simulink model "dynamic_calib"  (Simulink 8.8)
settings: Solver=FixedStepDiscrete  StartTime=0.0  StopTime=tEnd  FixedStep=CONFIG.Ts  RelTol=1e-3  EnableMultiTasking=on
undefined symbols (not defined in the file or in its folder): calibDelta, CONFIG, tSwitch, USE_h_ONLY, USE_JOINT_VELOCITY
libraries: WBToolboxLibrary x32
settings Model: SuppressorTable=22 serialization::archive 11 0 3 0 0 0 11 0  Creator=gabri  LastModifiedBy=gnava
settings DataIOCC: SignalLoggingSaveFormat=Dataset
settings DebuggingCC: UnderspecifiedInitializationDetection=Simplified  MergeDetectMultiDrivingBlocksExec=error  SolverPrmCheckMsg=warning  FcnCallInpInsideContextMsg=error  StateNameClashWarn=none
settings GRTTargetCC: CombineOutputUpdateFcns=on  GRTInterface=off
settings ConfigComp: CovSFcnEnable=off

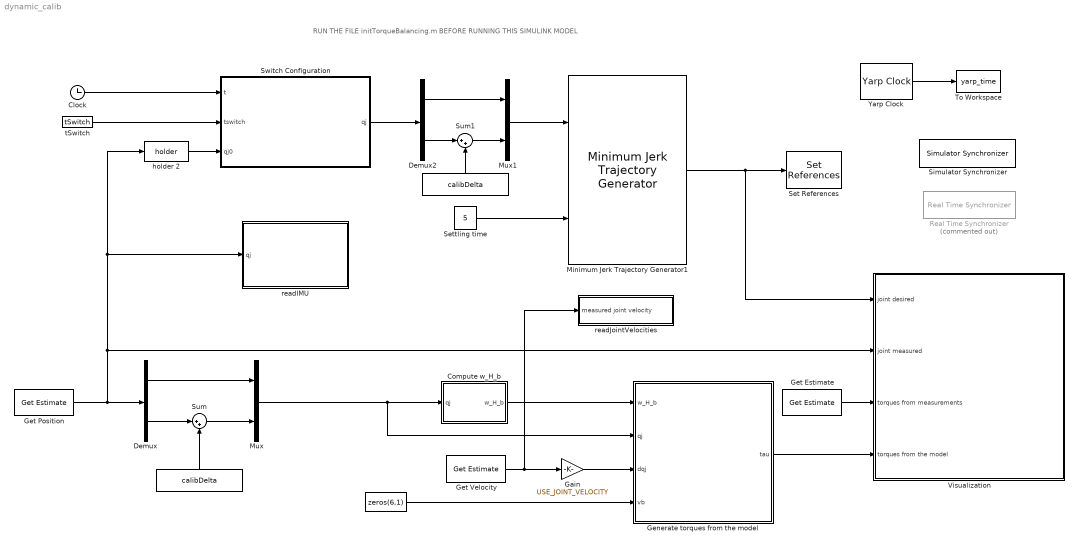
== system dynamic_calib ==
  note: RUN THE FILE initTorqueBalancing.m BEFORE RUNNING THIS SIMULINK MODEL
  "           " : Constant  Value=zeros(6,1)
  "                   " : Constant  Value=calibDelta
  "                                                      " : Constant  Value=calibDelta
  Clock : Clock
  Compute w_H_b : Subsystem
  Demux : Demux  Outputs=[13;12]
  Demux2 : Demux  Outputs=[13;12]
  Gain : Gain  Gain=USE_JOINT_VELOCITY
  Generate torques from the model : Subsystem
  Get Estimate : WBToolboxLibrary/wholeBodyStates/Get Estimate  estimateType=Joints Torque  robotName=WBT_robotName  localName=WBT_modelName  wbiFile=WBT_wbiFilename  wbiList=WBT_wbiList
  Get Position : WBToolboxLibrary/wholeBodyStates/Get Estimate  estimateType=Joints Position  robotName=WBT_robotName  localName=WBT_modelName  wbiFile=WBT_wbiFilename  wbiList=WBT_wbiList
  Get Velocity : WBToolboxLibrary/wholeBodyStates/Get Estimate  estimateType=Joints Velocity  robotName=WBT_robotName  localName=WBT_modelName  wbiFile=WBT_wbiFilename  wbiList=WBT_wbiList
  Minimum Jerk Trajectory Generator1 : WBToolboxLibrary/Utilities/Minimum Jerk Trajectory Generator  externalSettlingTime=on  settlingTime=1  sampleTime=CONFIG.Ts  resetOnSettlingTime=off  firstDerivatives=off  secondDerivatives=off  explicitInitialValue=off
  Mux : Mux  Inputs=2
  Mux1 : Mux  Inputs=2
  Real Time Synchronizer : WBToolboxLibrary/Utilities/Real Time Synchronizer  Commented=on  period=0.01
  Set References : WBToolboxLibrary/wholeBodyActuators/Set References  controlType=Position Direct  fullOrSubControl=Full  controlledJoints=''  robotName=WBT_robotName  localName=WBT_modelName  wbiFile=WBT_wbiFilename  wbiList=WBT_wbiList
  Settling time : Constant  Value=5
  Simulator Synchronizer : WBToolboxLibrary/Utilities/Simulator Synchronizer  period=0.01  serverPortName='/clock/rpc'  clientPortName='/WBT_synchronizer/rpc:o'
  Sum : Sum  Inputs=|++
  Sum1 : Sum  Inputs=|++
  Switch Configuration : MATLAB Function  TreatAsAtomicUnit=on
  To Workspace : ToWorkspace  VariableName=yarp_time  SaveFormat=Structure With Time  SampleTime=-1
  Visualization : Subsystem
  Yarp Clock : WBToolboxLibrary/Utilities/Yarp Clock
  holder 2 : WBToolboxLibrary/Utilities/holder 
  readIMU : Subsystem
  readJointVelocities : Subsystem
  tSwitch : Constant  Value=tSwitch
  wires:
  "                                                      "/1 -> Sum/2
  Get Estimate/1 -> Visualization/3(torques from measurements)
  Get Position/1 -> readIMU/1(qj), holder 2/1, Visualization/2("joint measured "), Demux/1
  Demux/2 -> Sum/1
  Demux/1 -> Mux/1
  Mux/1 -> Generate torques from the model/2(qj), Compute w_H_b/1(qj)
  Sum/1 -> Mux/2
  Settling time/1 -> Minimum Jerk Trajectory Generator1/2
  Clock/1 -> Switch Configuration/1(t)
  tSwitch/1 -> Switch Configuration/2(tswitch)
  holder 2/1 -> Switch Configuration/3(qj0)
  Get Velocity/1 -> readJointVelocities/1("measured joint velocity "), Gain/1
  "           "/1 -> Generate torques from the model/4(vb)
  Generate torques from the model/1(tau) -> Visualization/4(torques from the model)
  "                   "/1 -> Sum1/2
  Switch Configuration/1(qj) -> Demux2/1
  Demux2/2 -> Sum1/1
  Demux2/1 -> Mux1/1
  Sum1/1 -> Mux1/2
  Mux1/1 -> Minimum Jerk Trajectory Generator1/1
  Minimum Jerk Trajectory Generator1/1 -> Visualization/1(joint desired), Set References/1
  Compute w_H_b/1(w_H_b) -> Generate torques from the model/1(w_H_b)
  Gain/1 -> Generate torques from the model/3(dqj)
  Yarp Clock/1 -> To Workspace/1

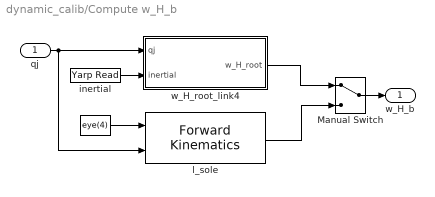
== system dynamic_calib/Compute w_H_b ==
  qj : Inport
  " " : Constant  Value=eye(4)
  Manual Switch : ManualSwitch
  inertial : WBToolboxLibrary/Utilities/Yarp Read  portName=PORTS.IMU_CALIB  signalSize=12  blocking=off  timestamp=off  autoconnect=on  errorOnConnection=on
  l_sole : WBToolboxLibrary/wholeBodyModel/Kinematics/Forward Kinematics  frameName='Waist'  robotName=WBT_robotName  localName=WBT_modelName  wbiFile=WBT_wbiFilename  wbiList=WBT_wbiList
  w_H_root_link4 : Subsystem  mask{link_name='Waist'}
      mask prompts: link_name "link name"
      mask help:
      | This block evaluates the homogeneous transformation between the world and the root link, i.e. ^wH_b. It assumes that the link specified by the variable 'link_name' has a constant position
      | w.r.t. an inertial frame, but it can rotate arbitrarily. This rotation is retrived from the IMU sensor.
      mask Display:
      | str = strrep(link_name, '_','\_');
      | port_label('output',1,['{}^{',str '}H_{root}'],'texmode','on')
      | clear str;
      | 
      | port_label('input',1,'q_j','texmode','on')
      | 
      | port_label('input',2,'inertial','texmode','on')
  w_H_b : Outport
  wires:
  qj/1 -> w_H_root_link4/1(qj), l_sole/2
  inertial/1 -> w_H_root_link4/2(inertial)
  " "/1 -> l_sole/1
  Manual Switch/1 -> w_H_b/1
  w_H_root_link4/1(w_H_root) -> Manual Switch/1
  l_sole/1 -> Manual Switch/2

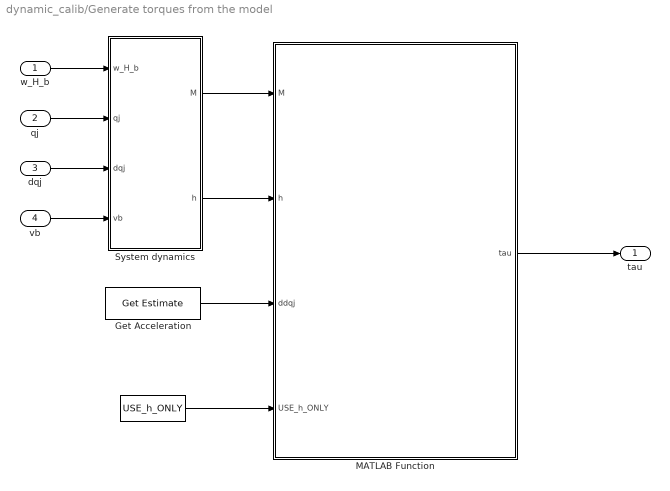
== system dynamic_calib/Generate torques from the model ==
  w_H_b : Inport
  qj : Inport  Port=2
  dqj : Inport  Port=3
  vb : Inport  Port=4
  "           " : Constant  Value=USE_h_ONLY
  Get Acceleration : WBToolboxLibrary/wholeBodyStates/Get Estimate  estimateType=Joints Acceleration  robotName=WBT_robotName  localName=WBT_modelName  wbiFile=WBT_wbiFilename  wbiList=WBT_wbiList
  MATLAB Function : MATLAB Function  TreatAsAtomicUnit=on
  System dynamics : Subsystem
  tau : Outport
  wires:
  qj/1 -> System dynamics/2(qj)
  w_H_b/1 -> System dynamics/1(w_H_b)
  MATLAB Function/1(tau) -> tau/1
  dqj/1 -> System dynamics/3(dqj)
  vb/1 -> System dynamics/4(vb)
  System dynamics/1("M ") -> MATLAB Function/1(M)
  System dynamics/2(h) -> MATLAB Function/2(h)
  Get Acceleration/1 -> MATLAB Function/3(ddqj)
  "           "/1 -> MATLAB Function/4(USE_h_ONLY)

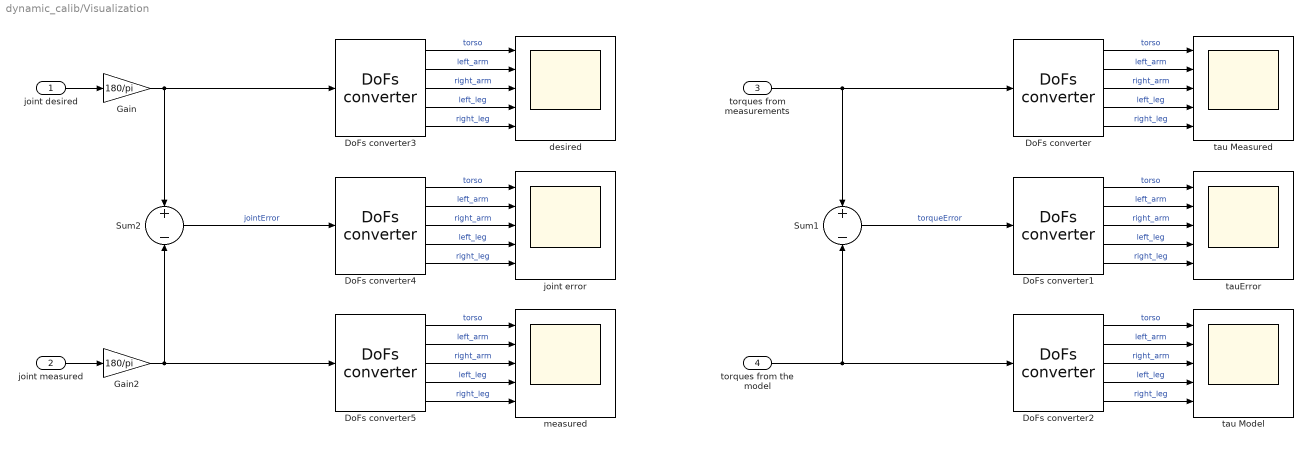
== system dynamic_calib/Visualization ==
  joint desired : Inport
  "joint measured " : Inport  Port=2
  torques from measurements : Inport  Port=3
  torques from the model : Inport  Port=4
  DoFs converter{,1..5} (6 alike) : WBToolboxLibrary/Utilities/DoFs converter  yarp2WBIOption=From WBI to YARP  robotName=WBT_robotName  localName=WBT_modelName  wbiFile=WBT_wbiFilename  wbiList=WBT_wbiList
  Gain : Gain  Gain=180/pi
  Gain2 : Gain  Gain=180/pi
  Sum1 : Sum  Inputs=+-
  Sum2 : Sum  Inputs=+-
  desired : Scope  NumInputPorts=5
  joint error : Scope  NumInputPorts=5
  measured : Scope  NumInputPorts=5
  tau Measured : Scope  NumInputPorts=5
  tau Model : Scope  NumInputPorts=5
  tauError : Scope  NumInputPorts=5
  wires:
  DoFs converter2/3 -> tau Model/3  "right_arm"
  torques from the model/1 -> DoFs converter2/1, Sum1/2
  DoFs converter/4 -> tau Measured/4  "left_leg"
  DoFs converter/3 -> tau Measured/3  "right_arm"
  DoFs converter1/5 -> tauError/5  "right_leg"
  DoFs converter1/1 -> tauError/1  "torso"
  DoFs converter1/2 -> tauError/2  "left_arm"
  DoFs converter1/4 -> tauError/4  "left_leg"
  DoFs converter1/3 -> tauError/3  "right_arm"
  Sum1/1 -> DoFs converter1/1  "torqueError"
  DoFs converter2/5 -> tau Model/5  "right_leg"
  DoFs converter2/1 -> tau Model/1  "torso"
  DoFs converter2/2 -> tau Model/2  "left_arm"
  DoFs converter2/4 -> tau Model/4  "left_leg"
  torques from measurements/1 -> DoFs converter/1, Sum1/1
  DoFs converter/5 -> tau Measured/5  "right_leg"
  DoFs converter/1 -> tau Measured/1  "torso"
  DoFs converter/2 -> tau Measured/2  "left_arm"
  DoFs converter5/3 -> measured/3  "right_arm"
  "joint measured "/1 -> Gain2/1
  DoFs converter3/4 -> desired/4  "left_leg"
  DoFs converter3/3 -> desired/3  "right_arm"
  DoFs converter4/5 -> joint error/5  "right_leg"
  DoFs converter4/1 -> joint error/1  "torso"
  DoFs converter4/2 -> joint error/2  "left_arm"
  DoFs converter4/4 -> joint error/4  "left_leg"
  DoFs converter4/3 -> joint error/3  "right_arm"
  Sum2/1 -> DoFs converter4/1  "jointError"
  DoFs converter5/5 -> measured/5  "right_leg"
  DoFs converter5/1 -> measured/1  "torso"
  DoFs converter5/2 -> measured/2  "left_arm"
  DoFs converter5/4 -> measured/4  "left_leg"
  joint desired/1 -> Gain/1
  DoFs converter3/5 -> desired/5  "right_leg"
  DoFs converter3/1 -> desired/1  "torso"
  DoFs converter3/2 -> desired/2  "left_arm"
  Gain/1 -> DoFs converter3/1, Sum2/1
  Gain2/1 -> DoFs converter5/1, Sum2/2

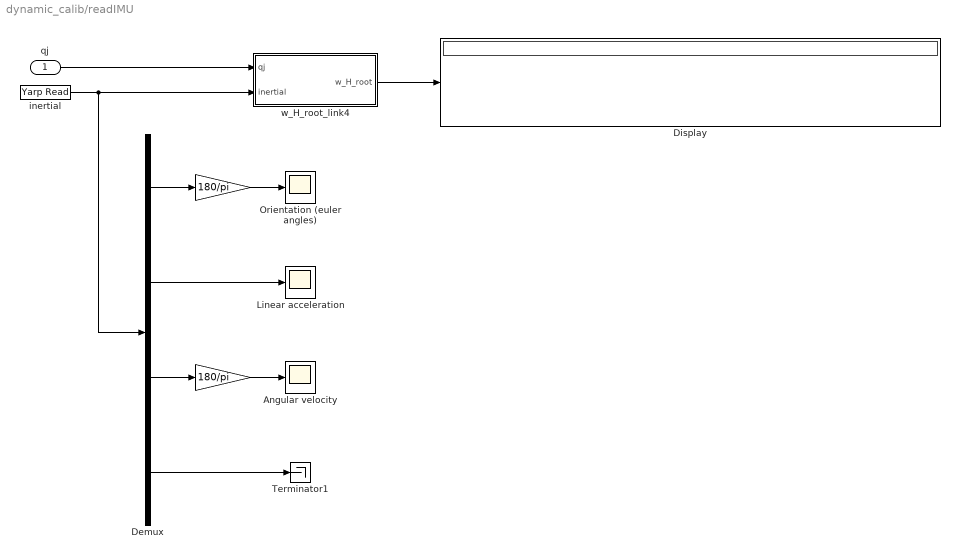
== system dynamic_calib/readIMU ==
  qj : Inport
  " " : Gain  Gain=180/pi
  "  " : Gain  Gain=180/pi
  Angular velocity : Scope
  Demux : Demux  Outputs=[3;3;3;3]
  Display : Display
  Linear acceleration : Scope
  Orientation (euler angles) : Scope
  Terminator1 : Terminator
  inertial : WBToolboxLibrary/Utilities/Yarp Read  portName=PORTS.IMU_CALIB  signalSize=12  blocking=off  timestamp=off  autoconnect=on  errorOnConnection=on
  w_H_root_link4 : Subsystem  mask{link_name='Waist'}
      mask prompts: link_name "link name"
      mask help:
      | This block evaluates the homogeneous transformation between the world and the root link, i.e. ^wH_b. It assumes that the link specified by the variable 'link_name' has a constant position
      | w.r.t. an inertial frame, but it can rotate arbitrarily. This rotation is retrived from the IMU sensor.
      mask Display:
      | str = strrep(link_name, '_','\_');
      | port_label('output',1,['{}^{',str '}H_{root}'],'texmode','on')
      | clear str;
      | 
      | port_label('input',1,'q_j','texmode','on')
      | 
      | port_label('input',2,'inertial','texmode','on')
  wires:
  qj/1 -> w_H_root_link4/1(qj)
  w_H_root_link4/1(w_H_root) -> Display/1
  Demux/1 -> "  "/1
  Demux/2 -> Linear acceleration/1
  Demux/3 -> " "/1
  inertial/1 -> w_H_root_link4/2(inertial), Demux/1
  Demux/4 -> Terminator1/1
  "  "/1 -> Orientation (euler angles)/1
  " "/1 -> Angular velocity/1

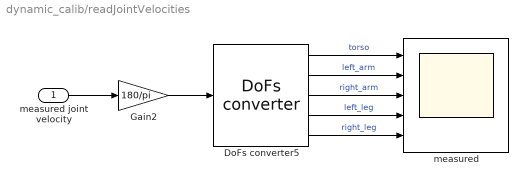
== system dynamic_calib/readJointVelocities ==
  "measured joint velocity " : Inport
  DoFs converter5 : WBToolboxLibrary/Utilities/DoFs converter  yarp2WBIOption=From WBI to YARP  robotName=WBT_robotName  localName=WBT_modelName  wbiFile=WBT_wbiFilename  wbiList=WBT_wbiList
  Gain2 : Gain  Gain=180/pi
  measured : Scope  NumInputPorts=5
  wires:
  DoFs converter5/3 -> measured/3  "right_arm"
  "measured joint velocity "/1 -> Gain2/1
  DoFs converter5/5 -> measured/5  "right_leg"
  DoFs converter5/1 -> measured/1  "torso"
  DoFs converter5/2 -> measured/2  "left_arm"
  DoFs converter5/4 -> measured/4  "left_leg"
  Gain2/1 -> DoFs converter5/1

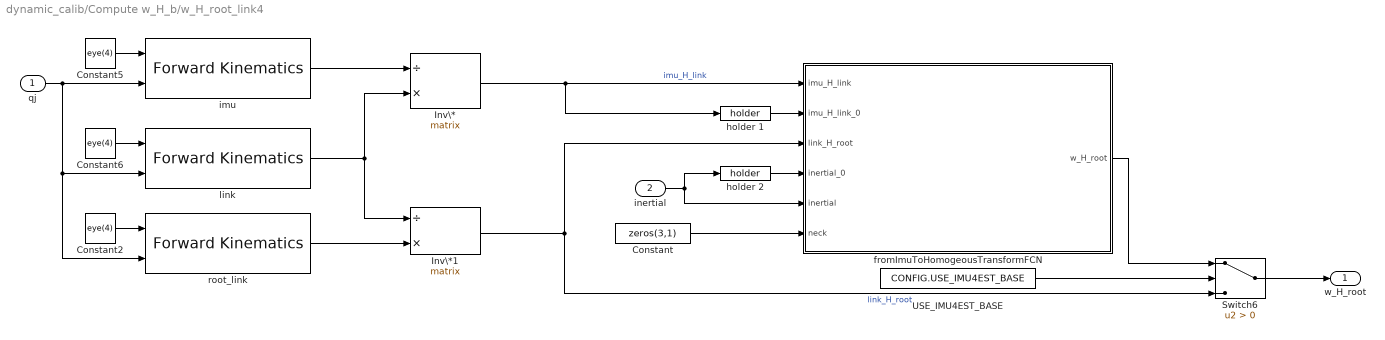
== system dynamic_calib/Compute w_H_b/w_H_root_link4 ==
  qj : Inport
  inertial : Inport  Port=2
  Constant : Constant  Value=zeros(3,1)
  Constant2 : Constant  Value=eye(4)
  Constant5 : Constant  Value=eye(4)
  Constant6 : Constant  Value=eye(4)
  Inv\* : Product  Inputs=/*  Multiplication=Matrix(*)
  Inv\*1 : Product  Inputs=/*  Multiplication=Matrix(*)
  Switch6 : Switch  Criteria=u2 > Threshold
  USE_IMU4EST_BASE : Constant  Value=CONFIG.USE_IMU4EST_BASE
  fromImuToHomogeousTransformFCN : MATLAB Function  TreatAsAtomicUnit=on
  holder 1 : WBToolboxLibrary/Utilities/holder 
  holder 2 : WBToolboxLibrary/Utilities/holder 
  imu : WBToolboxLibrary/wholeBodyModel/Kinematics/Forward Kinematics  frameName=FRAMES.IMU  robotName=WBT_robotName  localName=WBT_modelName  wbiFile=WBT_wbiFilename  wbiList=WBT_wbiList
  link : WBToolboxLibrary/wholeBodyModel/Kinematics/Forward Kinematics  frameName=link_name  robotName=WBT_robotName  localName=WBT_modelName  wbiFile=WBT_wbiFilename  wbiList=WBT_wbiList
  root_link : WBToolboxLibrary/wholeBodyModel/Kinematics/Forward Kinematics  frameName=FRAMES.BASE  robotName=WBT_robotName  localName=WBT_modelName  wbiFile=WBT_wbiFilename  wbiList=WBT_wbiList
  w_H_root : Outport
  wires:
  Constant5/1 -> imu/1
  Inv\*/1 -> holder 1/1, fromImuToHomogeousTransformFCN/1(imu_H_link)  "imu_H_link"
  imu/1 -> Inv\*/1
  Constant6/1 -> link/1
  Inv\*1/1 -> Switch6/3, fromImuToHomogeousTransformFCN/3(link_H_root)  "link_H_root"
  link/1 -> Inv\*/2, Inv\*1/1
  inertial/1 -> holder 2/1, fromImuToHomogeousTransformFCN/5(inertial)
  Switch6/1 -> w_H_root/1
  USE_IMU4EST_BASE/1 -> Switch6/2
  fromImuToHomogeousTransformFCN/1(w_H_root) -> Switch6/1
  Constant2/1 -> root_link/1
  qj/1 -> root_link/2, link/2, imu/2
  root_link/1 -> Inv\*1/2
  holder 1/1 -> fromImuToHomogeousTransformFCN/2(imu_H_link_0)
  holder 2/1 -> fromImuToHomogeousTransformFCN/4(inertial_0)
  Constant/1 -> fromImuToHomogeousTransformFCN/6(neck)

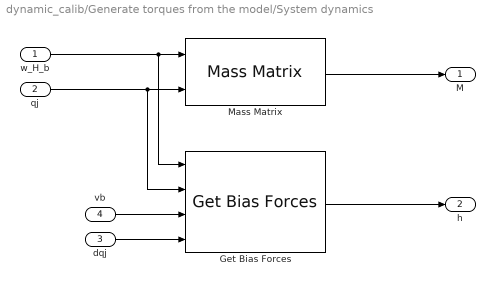
== system dynamic_calib/Generate torques from the model/System dynamics ==
  w_H_b : Inport
  qj : Inport  Port=2
  dqj : Inport  Port=3
  vb : Inport  Port=4
  Get Bias Forces : WBToolboxLibrary/wholeBodyModel/Dynamics/Get Bias Forces  robotName=WBT_robotName  localName=WBT_modelName  wbiFile=WBT_wbiFilename  wbiList=WBT_wbiList  explicitGravity=off
  Mass Matrix : WBToolboxLibrary/wholeBodyModel/Dynamics/Mass Matrix  robotName=WBT_robotName  localName=WBT_modelName  wbiFile=WBT_wbiFilename  wbiList=WBT_wbiList
  "M " : Outport
  h : Outport  Port=2
  wires:
  Mass Matrix/1 -> "M "/1
  Get Bias Forces/1 -> h/1
  w_H_b/1 -> Get Bias Forces/1, Mass Matrix/1
  qj/1 -> Get Bias Forces/2, Mass Matrix/2
  vb/1 -> Get Bias Forces/3
  dqj/1 -> Get Bias Forces/4

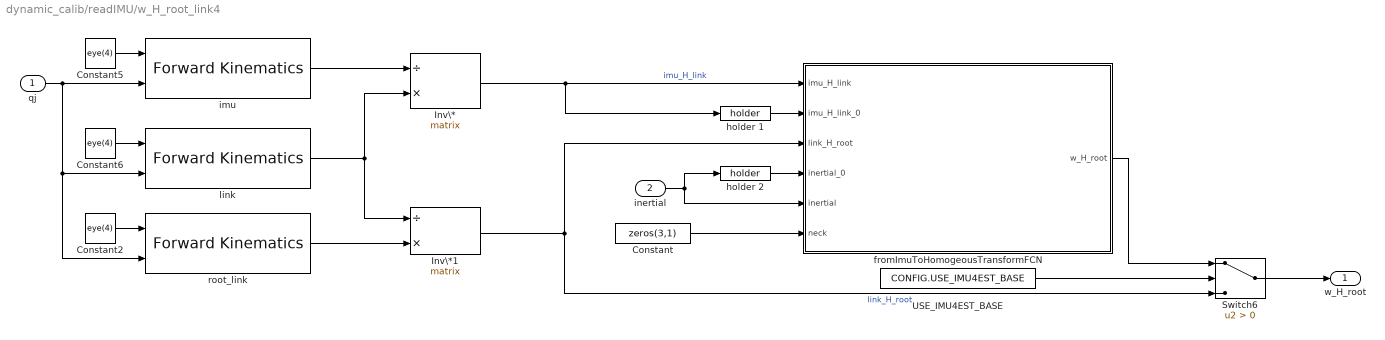
== system dynamic_calib/readIMU/w_H_root_link4 ==
  qj : Inport
  inertial : Inport  Port=2
  Constant : Constant  Value=zeros(3,1)
  Constant2 : Constant  Value=eye(4)
  Constant5 : Constant  Value=eye(4)
  Constant6 : Constant  Value=eye(4)
  Inv\* : Product  Inputs=/*  Multiplication=Matrix(*)
  Inv\*1 : Product  Inputs=/*  Multiplication=Matrix(*)
  Switch6 : Switch  Criteria=u2 > Threshold
  USE_IMU4EST_BASE : Constant  Value=CONFIG.USE_IMU4EST_BASE
  fromImuToHomogeousTransformFCN : MATLAB Function  TreatAsAtomicUnit=on
  holder 1 : WBToolboxLibrary/Utilities/holder 
  holder 2 : WBToolboxLibrary/Utilities/holder 
  imu : WBToolboxLibrary/wholeBodyModel/Kinematics/Forward Kinematics  frameName=FRAMES.IMU  robotName=WBT_robotName  localName=WBT_modelName  wbiFile=WBT_wbiFilename  wbiList=WBT_wbiList
  link : WBToolboxLibrary/wholeBodyModel/Kinematics/Forward Kinematics  frameName=link_name  robotName=WBT_robotName  localName=WBT_modelName  wbiFile=WBT_wbiFilename  wbiList=WBT_wbiList
  root_link : WBToolboxLibrary/wholeBodyModel/Kinematics/Forward Kinematics  frameName=FRAMES.BASE  robotName=WBT_robotName  localName=WBT_modelName  wbiFile=WBT_wbiFilename  wbiList=WBT_wbiList
  w_H_root : Outport
  wires:
  Constant5/1 -> imu/1
  Inv\*/1 -> holder 1/1, fromImuToHomogeousTransformFCN/1(imu_H_link)  "imu_H_link"
  imu/1 -> Inv\*/1
  Constant6/1 -> link/1
  Inv\*1/1 -> Switch6/3, fromImuToHomogeousTransformFCN/3(link_H_root)  "link_H_root"
  link/1 -> Inv\*/2, Inv\*1/1
  inertial/1 -> holder 2/1, fromImuToHomogeousTransformFCN/5(inertial)
  Switch6/1 -> w_H_root/1
  USE_IMU4EST_BASE/1 -> Switch6/2
  fromImuToHomogeousTransformFCN/1(w_H_root) -> Switch6/1
  Constant2/1 -> root_link/1
  qj/1 -> root_link/2, link/2, imu/2
  root_link/1 -> Inv\*1/2
  holder 1/1 -> fromImuToHomogeousTransformFCN/2(imu_H_link_0)
  holder 2/1 -> fromImuToHomogeousTransformFCN/4(inertial_0)
  Constant/1 -> fromImuToHomogeousTransformFCN/6(neck)

== matlab function Generate torques from the model/MATLAB Function ==
  data: M input double; tau output double; h input double; ddqj input double; USE_h_ONLY input double
function tau = computeForwardDynamicsFCN(M,h,ddqj,USE_h_ONLY)

    tau = computeForwardDynamics(M,h,ddqj,USE_h_ONLY);

end

== matlab function Switch Configuration ==
  data: t input double; qj output double; tswitch input double; qj0 input double; CONFIG parameter double
function qj = changeConfigFCN(t,tswitch,qj0,CONFIG)

qj = changeConfig(t,tswitch,qj0,CONFIG);

end

== matlab function readIMU/w_H_root_link4/fromImuToHomogeousTransformFCN ==
  data: imu_H_link input double; imu_H_link_0 input double; link_H_root input double; inertial_0 input double; inertial input double; neck input double; w_H_root output double; CONFIG parameter double
function w_H_root = fromBaseToWorldWithImuFCN(imu_H_link,imu_H_link_0,link_H_root,inertial_0,inertial,neck,CONFIG)

w_H_root = fromBaseToWorldWithImu(imu_H_link,imu_H_link_0,link_H_root,inertial_0,inertial,neck,CONFIG);

end

== matlab function Compute w_H_b/w_H_root_link4/fromImuToHomogeousTransformFCN ==
  data: imu_H_link input double; imu_H_link_0 input double; link_H_root input double; inertial_0 input double; inertial input double; neck input double; w_H_root output double; CONFIG parameter double
function w_H_root = fromBaseToWorldWithImuFCN(imu_H_link,imu_H_link_0,link_H_root,inertial_0,inertial,neck,CONFIG)

w_H_root = fromBaseToWorldWithImu(imu_H_link,imu_H_link_0,link_H_root,inertial_0,inertial,neck,CONFIG);

end
